simulink model "Water_Treatment_Plant"  (R2026a)
settings: Solver=ode4  StopTime=P.sim.defaultStopTime_s  FixedStep=P.sim.baseStep_s
undefined symbols (not defined in the file): P
settings Model: Creator=jonat  LastModifiedBy=jonat

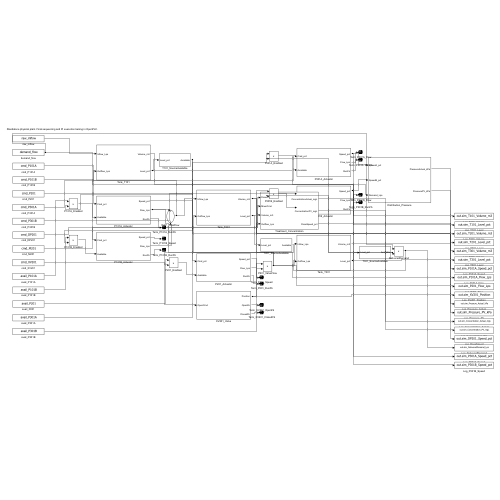
[thumbnail: Simulink's stored preview of the top-level diagram]
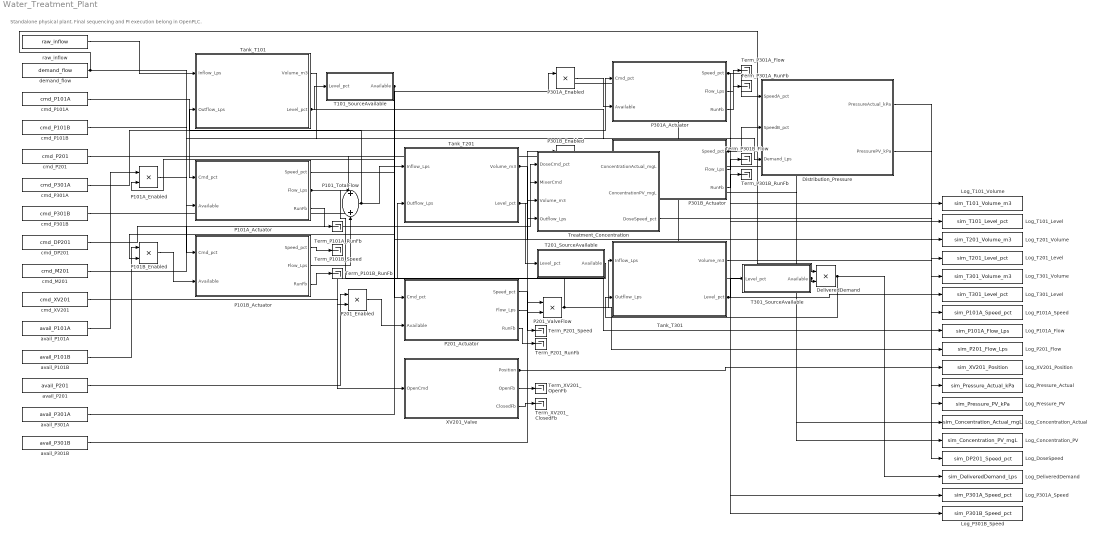
== system Water_Treatment_Plant ==
  note: Standalone physical plant. Final sequencing and PI execution belong in OpenPLC.
  DeliveredDemand : Product  Inputs=**
  Distribution_Pressure : Subsystem
  Log_Concentration_Actual : ToWorkspace  VariableName=sim_Concentration_Actual_mgL  SaveFormat=Timeseries  SampleTime=-1
  Log_Concentration_PV : ToWorkspace  VariableName=sim_Concentration_PV_mgL  SaveFormat=Timeseries  SampleTime=-1
  Log_DeliveredDemand : ToWorkspace  VariableName=sim_DeliveredDemand_Lps  SaveFormat=Timeseries  SampleTime=-1
  Log_DoseSpeed : ToWorkspace  VariableName=sim_DP201_Speed_pct  SaveFormat=Timeseries  SampleTime=-1
  Log_P101A_Flow : ToWorkspace  VariableName=sim_P101A_Flow_Lps  SaveFormat=Timeseries  SampleTime=-1
  Log_P101A_Speed : ToWorkspace  VariableName=sim_P101A_Speed_pct  SaveFormat=Timeseries  SampleTime=-1
  Log_P201_Flow : ToWorkspace  VariableName=sim_P201_Flow_Lps  SaveFormat=Timeseries  SampleTime=-1
  Log_P301A_Speed : ToWorkspace  VariableName=sim_P301A_Speed_pct  SaveFormat=Timeseries  SampleTime=-1
  Log_P301B_Speed : ToWorkspace  VariableName=sim_P301B_Speed_pct  SaveFormat=Timeseries  SampleTime=-1
  Log_Pressure_Actual : ToWorkspace  VariableName=sim_Pressure_Actual_kPa  SaveFormat=Timeseries  SampleTime=-1
  Log_Pressure_PV : ToWorkspace  VariableName=sim_Pressure_PV_kPa  SaveFormat=Timeseries  SampleTime=-1
  Log_T101_Level : ToWorkspace  VariableName=sim_T101_Level_pct  SaveFormat=Timeseries  SampleTime=-1
  Log_T101_Volume : ToWorkspace  VariableName=sim_T101_Volume_m3  SaveFormat=Timeseries  SampleTime=-1
  Log_T201_Level : ToWorkspace  VariableName=sim_T201_Level_pct  SaveFormat=Timeseries  SampleTime=-1
  Log_T201_Volume : ToWorkspace  VariableName=sim_T201_Volume_m3  SaveFormat=Timeseries  SampleTime=-1
  Log_T301_Level : ToWorkspace  VariableName=sim_T301_Level_pct  SaveFormat=Timeseries  SampleTime=-1
  Log_T301_Volume : ToWorkspace  VariableName=sim_T301_Volume_m3  SaveFormat=Timeseries  SampleTime=-1
  Log_XV201_Position : ToWorkspace  VariableName=sim_XV201_Position  SaveFormat=Timeseries  SampleTime=-1
  P101A_Actuator : Subsystem
  P101A_Enabled : Product  Inputs=**
  P101B_Actuator : Subsystem
  P101B_Enabled : Product  Inputs=**
  P101_TotalFlow : Sum
  P201_Actuator : Subsystem
  P201_Enabled : Product  Inputs=**
  P201_ValveFlow : Product  Inputs=**
  P301A_Actuator : Subsystem
  P301A_Enabled : Product  Inputs=**
  P301B_Actuator : Subsystem
  P301B_Enabled : Product  Inputs=**
  T101_SourceAvailable : Subsystem
  T201_SourceAvailable : Subsystem
  T301_SourceAvailable : Subsystem
  Tank_T101 : Subsystem
  Tank_T201 : Subsystem
  Tank_T301 : Subsystem
  Term_P101A_RunFb : Terminator
  Term_P101B_RunFb : Terminator
  Term_P101B_Speed : Terminator
  Term_P201_RunFb : Terminator
  Term_P201_Speed : Terminator
  Term_P301A_Flow : Terminator
  Term_P301A_RunFb : Terminator
  Term_P301B_Flow : Terminator
  Term_P301B_RunFb : Terminator
  Term_XV201_ClosedFb : Terminator
  Term_XV201_OpenFb : Terminator
  Treatment_Concentration : Subsystem
  XV201_Valve : Subsystem
  avail_P101A : FromWorkspace  VariableName=avail_P101A  Interpolate=off  OutputAfterFinalValue=Holding final value
  avail_P101B : FromWorkspace  VariableName=avail_P101B  Interpolate=off  OutputAfterFinalValue=Holding final value
  avail_P201 : FromWorkspace  VariableName=avail_P201  Interpolate=off  OutputAfterFinalValue=Holding final value
  avail_P301A : FromWorkspace  VariableName=avail_P301A  Interpolate=off  OutputAfterFinalValue=Holding final value
  avail_P301B : FromWorkspace  VariableName=avail_P301B  Interpolate=off  OutputAfterFinalValue=Holding final value
  cmd_DP201 : FromWorkspace  VariableName=cmd_DP201  Interpolate=off  OutputAfterFinalValue=Holding final value
  cmd_M201 : FromWorkspace  VariableName=cmd_M201  Interpolate=off  OutputAfterFinalValue=Holding final value
  cmd_P101A : FromWorkspace  VariableName=cmd_P101A  Interpolate=off  OutputAfterFinalValue=Holding final value
  cmd_P101B : FromWorkspace  VariableName=cmd_P101B  Interpolate=off  OutputAfterFinalValue=Holding final value
  cmd_P201 : FromWorkspace  VariableName=cmd_P201  Interpolate=off  OutputAfterFinalValue=Holding final value
  cmd_P301A : FromWorkspace  VariableName=cmd_P301A  Interpolate=off  OutputAfterFinalValue=Holding final value
  cmd_P301B : FromWorkspace  VariableName=cmd_P301B  Interpolate=off  OutputAfterFinalValue=Holding final value
  cmd_XV201 : FromWorkspace  VariableName=cmd_XV201  Interpolate=off  OutputAfterFinalValue=Holding final value
  demand_flow : FromWorkspace  VariableName=demand_flow  Interpolate=off  OutputAfterFinalValue=Holding final value
  raw_inflow : FromWorkspace  VariableName=raw_inflow  Interpolate=off  OutputAfterFinalValue=Holding final value
  wires:
  raw_inflow/1 -> Tank_T101/1(Inflow_Lps)
  Tank_T101/2(Level_pct) -> T101_SourceAvailable/1(Level_pct), Log_T101_Level/1
  avail_P101A/1 -> P101A_Enabled/1
  T101_SourceAvailable/1(Available) -> P101A_Enabled/2, P101B_Enabled/2
  avail_P101B/1 -> P101B_Enabled/1
  cmd_P101A/1 -> P101A_Actuator/1(Cmd_pct)
  P101A_Enabled/1 -> P101A_Actuator/2(Available)
  cmd_P101B/1 -> P101B_Actuator/1(Cmd_pct)
  P101B_Enabled/1 -> P101B_Actuator/2(Available)
  P101A_Actuator/2(Flow_Lps) -> P101_TotalFlow/1, Log_P101A_Flow/1
  P101B_Actuator/2(Flow_Lps) -> P101_TotalFlow/2
  P101_TotalFlow/1 -> Tank_T101/2(Outflow_Lps), Tank_T201/1(Inflow_Lps)
  Tank_T201/2(Level_pct) -> T201_SourceAvailable/1(Level_pct), Log_T201_Level/1
  avail_P201/1 -> P201_Enabled/1
  T201_SourceAvailable/1(Available) -> P201_Enabled/2
  cmd_P201/1 -> P201_Actuator/1(Cmd_pct)
  P201_Enabled/1 -> P201_Actuator/2(Available)
  cmd_XV201/1 -> XV201_Valve/1(OpenCmd)
  P201_Actuator/2(Flow_Lps) -> P201_ValveFlow/1
  XV201_Valve/1(Position) -> P201_ValveFlow/2, Log_XV201_Position/1
  P201_ValveFlow/1 -> Tank_T201/2(Outflow_Lps), Tank_T301/1(Inflow_Lps), Treatment_Concentration/4(Outflow_Lps), Log_P201_Flow/1
  cmd_DP201/1 -> Treatment_Concentration/1(DoseCmd_pct)
  cmd_M201/1 -> Treatment_Concentration/2(MixerCmd)
  Tank_T201/1(Volume_m3) -> Treatment_Concentration/3(Volume_m3), Log_T201_Volume/1
  Tank_T301/2(Level_pct) -> T301_SourceAvailable/1(Level_pct), Log_T301_Level/1
  demand_flow/1 -> DeliveredDemand/1, Distribution_Pressure/3(Demand_Lps)
  T301_SourceAvailable/1(Available) -> DeliveredDemand/2, P301A_Enabled/2, P301B_Enabled/2
  DeliveredDemand/1 -> Tank_T301/2(Outflow_Lps), Log_DeliveredDemand/1
  avail_P301A/1 -> P301A_Enabled/1
  avail_P301B/1 -> P301B_Enabled/1
  cmd_P301A/1 -> P301A_Actuator/1(Cmd_pct)
  P301A_Enabled/1 -> P301A_Actuator/2(Available)
  cmd_P301B/1 -> P301B_Actuator/1(Cmd_pct)
  P301B_Enabled/1 -> P301B_Actuator/2(Available)
  P301A_Actuator/1(Speed_pct) -> Distribution_Pressure/1(SpeedA_pct), Log_P301A_Speed/1
  P301B_Actuator/1(Speed_pct) -> Distribution_Pressure/2(SpeedB_pct), Log_P301B_Speed/1
  P101A_Actuator/3(RunFb) -> Term_P101A_RunFb/1
  P101B_Actuator/1(Speed_pct) -> Term_P101B_Speed/1
  P101B_Actuator/3(RunFb) -> Term_P101B_RunFb/1
  P201_Actuator/1(Speed_pct) -> Term_P201_Speed/1
  P201_Actuator/3(RunFb) -> Term_P201_RunFb/1
  P301A_Actuator/2(Flow_Lps) -> Term_P301A_Flow/1
  P301A_Actuator/3(RunFb) -> Term_P301A_RunFb/1
  P301B_Actuator/2(Flow_Lps) -> Term_P301B_Flow/1
  P301B_Actuator/3(RunFb) -> Term_P301B_RunFb/1
  XV201_Valve/2(OpenFb) -> Term_XV201_OpenFb/1
  XV201_Valve/3(ClosedFb) -> Term_XV201_ClosedFb/1
  Tank_T101/1(Volume_m3) -> Log_T101_Volume/1
  Tank_T301/1(Volume_m3) -> Log_T301_Volume/1
  P101A_Actuator/1(Speed_pct) -> Log_P101A_Speed/1
  Distribution_Pressure/1(PressureActual_kPa) -> Log_Pressure_Actual/1
  Distribution_Pressure/2(PressurePV_kPa) -> Log_Pressure_PV/1
  Treatment_Concentration/1(ConcentrationActual_mgL) -> Log_Concentration_Actual/1
  Treatment_Concentration/2(ConcentrationPV_mgL) -> Log_Concentration_PV/1
  Treatment_Concentration/3(DoseSpeed_pct) -> Log_DoseSpeed/1

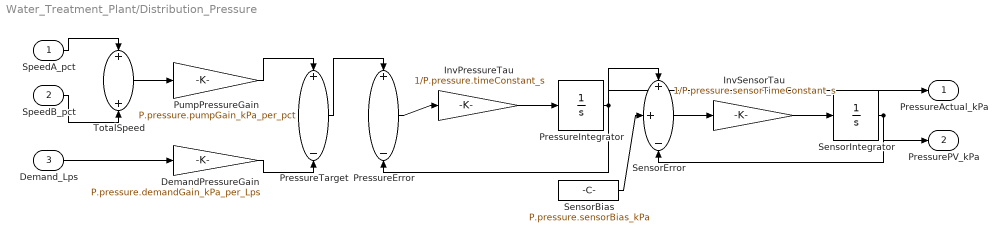
== system Water_Treatment_Plant/Distribution_Pressure ==
  SpeedA_pct : Inport
  SpeedB_pct : Inport  Port=2
  Demand_Lps : Inport  Port=3
  DemandPressureGain : Gain  Gain=P.pressure.demandGain_kPa_per_Lps
  InvPressureTau : Gain  Gain=1/P.pressure.timeConstant_s
  InvSensorTau : Gain  Gain=1/P.pressure.sensorTimeConstant_s
  PressureError : Sum  Inputs=+-
  PressureIntegrator : Integrator  InitialCondition=P.pressure.initial_kPa  LimitOutput=on  UpperSaturationLimit=P.sim.maxPressure_kPa  LowerSaturationLimit=0
  PressureTarget : Sum  Inputs=+-
  PumpPressureGain : Gain  Gain=P.pressure.pumpGain_kPa_per_pct
  SensorBias : Constant  Value=P.pressure.sensorBias_kPa
  SensorError : Sum  Inputs=++-
  SensorIntegrator : Integrator  InitialCondition=P.pressure.initial_kPa  LimitOutput=on  UpperSaturationLimit=P.sim.maxPressure_kPa  LowerSaturationLimit=0
  TotalSpeed : Sum
  PressureActual_kPa : Outport
  PressurePV_kPa : Outport  Port=2
  wires:
  SpeedA_pct/1 -> TotalSpeed/1
  SpeedB_pct/1 -> TotalSpeed/2
  TotalSpeed/1 -> PumpPressureGain/1
  Demand_Lps/1 -> DemandPressureGain/1
  PumpPressureGain/1 -> PressureTarget/1
  DemandPressureGain/1 -> PressureTarget/2
  PressureTarget/1 -> PressureError/1
  PressureIntegrator/1 -> PressureError/2, PressureActual_kPa/1, SensorError/1
  PressureError/1 -> InvPressureTau/1
  InvPressureTau/1 -> PressureIntegrator/1
  SensorBias/1 -> SensorError/2
  SensorIntegrator/1 -> SensorError/3, PressurePV_kPa/1
  SensorError/1 -> InvSensorTau/1
  InvSensorTau/1 -> SensorIntegrator/1

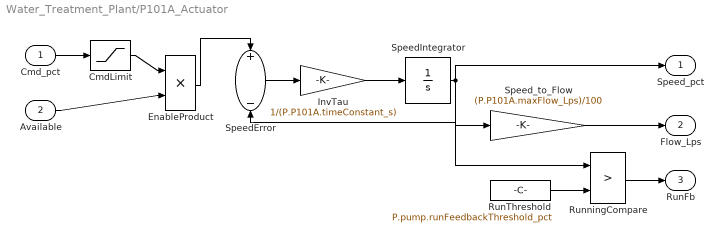
== system Water_Treatment_Plant/P101A_Actuator ==
  Cmd_pct : Inport
  Available : Inport  Port=2
  CmdLimit : Saturate  UpperLimit=100  LowerLimit=0
  EnableProduct : Product  Inputs=**
  InvTau : Gain  Gain=1/(P.P101A.timeConstant_s)
  RunThreshold : Constant  Value=P.pump.runFeedbackThreshold_pct
  RunningCompare : RelationalOperator  Operator=>  OutDataTypeStr=boolean  RndMeth=Simplest  InputSameDT=off
  SpeedError : Sum  Inputs=+-
  SpeedIntegrator : Integrator  LimitOutput=on  UpperSaturationLimit=100  LowerSaturationLimit=0
  Speed_to_Flow : Gain  Gain=(P.P101A.maxFlow_Lps)/100
  Speed_pct : Outport
  Flow_Lps : Outport  Port=2
  RunFb : Outport  Port=3
  wires:
  Cmd_pct/1 -> CmdLimit/1
  CmdLimit/1 -> EnableProduct/1
  Available/1 -> EnableProduct/2
  EnableProduct/1 -> SpeedError/1
  SpeedIntegrator/1 -> SpeedError/2, Speed_pct/1, Speed_to_Flow/1, RunningCompare/1
  SpeedError/1 -> InvTau/1
  InvTau/1 -> SpeedIntegrator/1
  Speed_to_Flow/1 -> Flow_Lps/1
  RunThreshold/1 -> RunningCompare/2
  RunningCompare/1 -> RunFb/1

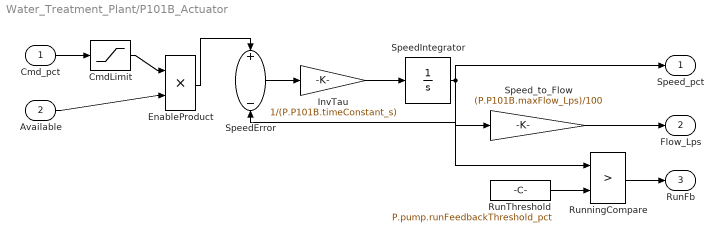
== system Water_Treatment_Plant/P101B_Actuator ==
  Cmd_pct : Inport
  Available : Inport  Port=2
  CmdLimit : Saturate  UpperLimit=100  LowerLimit=0
  EnableProduct : Product  Inputs=**
  InvTau : Gain  Gain=1/(P.P101B.timeConstant_s)
  RunThreshold : Constant  Value=P.pump.runFeedbackThreshold_pct
  RunningCompare : RelationalOperator  Operator=>  OutDataTypeStr=boolean  RndMeth=Simplest  InputSameDT=off
  SpeedError : Sum  Inputs=+-
  SpeedIntegrator : Integrator  LimitOutput=on  UpperSaturationLimit=100  LowerSaturationLimit=0
  Speed_to_Flow : Gain  Gain=(P.P101B.maxFlow_Lps)/100
  Speed_pct : Outport
  Flow_Lps : Outport  Port=2
  RunFb : Outport  Port=3
  wires:
  Cmd_pct/1 -> CmdLimit/1
  CmdLimit/1 -> EnableProduct/1
  Available/1 -> EnableProduct/2
  EnableProduct/1 -> SpeedError/1
  SpeedIntegrator/1 -> SpeedError/2, Speed_pct/1, Speed_to_Flow/1, RunningCompare/1
  SpeedError/1 -> InvTau/1
  InvTau/1 -> SpeedIntegrator/1
  Speed_to_Flow/1 -> Flow_Lps/1
  RunThreshold/1 -> RunningCompare/2
  RunningCompare/1 -> RunFb/1

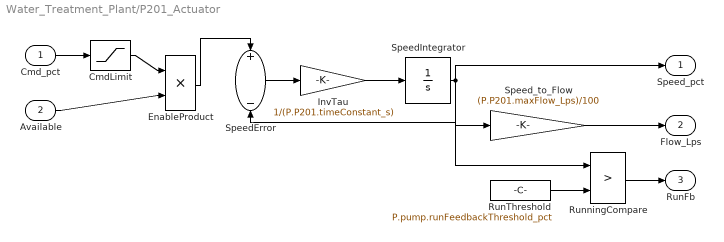
== system Water_Treatment_Plant/P201_Actuator ==
  Cmd_pct : Inport
  Available : Inport  Port=2
  CmdLimit : Saturate  UpperLimit=100  LowerLimit=0
  EnableProduct : Product  Inputs=**
  InvTau : Gain  Gain=1/(P.P201.timeConstant_s)
  RunThreshold : Constant  Value=P.pump.runFeedbackThreshold_pct
  RunningCompare : RelationalOperator  Operator=>  OutDataTypeStr=boolean  RndMeth=Simplest  InputSameDT=off
  SpeedError : Sum  Inputs=+-
  SpeedIntegrator : Integrator  LimitOutput=on  UpperSaturationLimit=100  LowerSaturationLimit=0
  Speed_to_Flow : Gain  Gain=(P.P201.maxFlow_Lps)/100
  Speed_pct : Outport
  Flow_Lps : Outport  Port=2
  RunFb : Outport  Port=3
  wires:
  Cmd_pct/1 -> CmdLimit/1
  CmdLimit/1 -> EnableProduct/1
  Available/1 -> EnableProduct/2
  EnableProduct/1 -> SpeedError/1
  SpeedIntegrator/1 -> SpeedError/2, Speed_pct/1, Speed_to_Flow/1, RunningCompare/1
  SpeedError/1 -> InvTau/1
  InvTau/1 -> SpeedIntegrator/1
  Speed_to_Flow/1 -> Flow_Lps/1
  RunThreshold/1 -> RunningCompare/2
  RunningCompare/1 -> RunFb/1

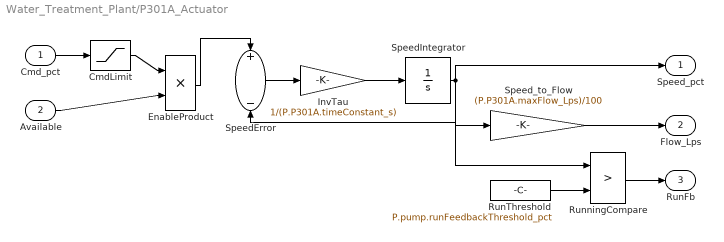
== system Water_Treatment_Plant/P301A_Actuator ==
  Cmd_pct : Inport
  Available : Inport  Port=2
  CmdLimit : Saturate  UpperLimit=100  LowerLimit=0
  EnableProduct : Product  Inputs=**
  InvTau : Gain  Gain=1/(P.P301A.timeConstant_s)
  RunThreshold : Constant  Value=P.pump.runFeedbackThreshold_pct
  RunningCompare : RelationalOperator  Operator=>  OutDataTypeStr=boolean  RndMeth=Simplest  InputSameDT=off
  SpeedError : Sum  Inputs=+-
  SpeedIntegrator : Integrator  LimitOutput=on  UpperSaturationLimit=100  LowerSaturationLimit=0
  Speed_to_Flow : Gain  Gain=(P.P301A.maxFlow_Lps)/100
  Speed_pct : Outport
  Flow_Lps : Outport  Port=2
  RunFb : Outport  Port=3
  wires:
  Cmd_pct/1 -> CmdLimit/1
  CmdLimit/1 -> EnableProduct/1
  Available/1 -> EnableProduct/2
  EnableProduct/1 -> SpeedError/1
  SpeedIntegrator/1 -> SpeedError/2, Speed_pct/1, Speed_to_Flow/1, RunningCompare/1
  SpeedError/1 -> InvTau/1
  InvTau/1 -> SpeedIntegrator/1
  Speed_to_Flow/1 -> Flow_Lps/1
  RunThreshold/1 -> RunningCompare/2
  RunningCompare/1 -> RunFb/1

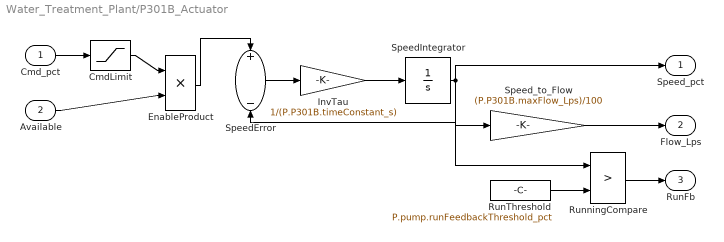
== system Water_Treatment_Plant/P301B_Actuator ==
  Cmd_pct : Inport
  Available : Inport  Port=2
  CmdLimit : Saturate  UpperLimit=100  LowerLimit=0
  EnableProduct : Product  Inputs=**
  InvTau : Gain  Gain=1/(P.P301B.timeConstant_s)
  RunThreshold : Constant  Value=P.pump.runFeedbackThreshold_pct
  RunningCompare : RelationalOperator  Operator=>  OutDataTypeStr=boolean  RndMeth=Simplest  InputSameDT=off
  SpeedError : Sum  Inputs=+-
  SpeedIntegrator : Integrator  LimitOutput=on  UpperSaturationLimit=100  LowerSaturationLimit=0
  Speed_to_Flow : Gain  Gain=(P.P301B.maxFlow_Lps)/100
  Speed_pct : Outport
  Flow_Lps : Outport  Port=2
  RunFb : Outport  Port=3
  wires:
  Cmd_pct/1 -> CmdLimit/1
  CmdLimit/1 -> EnableProduct/1
  Available/1 -> EnableProduct/2
  EnableProduct/1 -> SpeedError/1
  SpeedIntegrator/1 -> SpeedError/2, Speed_pct/1, Speed_to_Flow/1, RunningCompare/1
  SpeedError/1 -> InvTau/1
  InvTau/1 -> SpeedIntegrator/1
  Speed_to_Flow/1 -> Flow_Lps/1
  RunThreshold/1 -> RunningCompare/2
  RunningCompare/1 -> RunFb/1

== system Water_Treatment_Plant/T101_SourceAvailable ==
  Level_pct : Inport
  Compare : RelationalOperator  Operator=>  OutDataTypeStr=boolean  RndMeth=Simplest  InputSameDT=off
  MinimumLevel : Constant  Value=P.tank.minimumSourceLevel_pct
  Available : Outport
  wires:
  Level_pct/1 -> Compare/1
  MinimumLevel/1 -> Compare/2
  Compare/1 -> Available/1

== system Water_Treatment_Plant/T201_SourceAvailable ==
  Level_pct : Inport
  Compare : RelationalOperator  Operator=>  OutDataTypeStr=boolean  RndMeth=Simplest  InputSameDT=off
  MinimumLevel : Constant  Value=P.tank.minimumSourceLevel_pct
  Available : Outport
  wires:
  Level_pct/1 -> Compare/1
  MinimumLevel/1 -> Compare/2
  Compare/1 -> Available/1

== system Water_Treatment_Plant/T301_SourceAvailable ==
  Level_pct : Inport
  Compare : RelationalOperator  Operator=>  OutDataTypeStr=boolean  RndMeth=Simplest  InputSameDT=off
  MinimumLevel : Constant  Value=P.tank.minimumSourceLevel_pct
  Available : Outport
  wires:
  Level_pct/1 -> Compare/1
  MinimumLevel/1 -> Compare/2
  Compare/1 -> Available/1

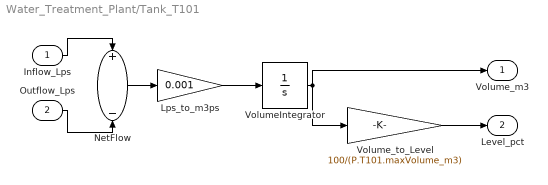
== system Water_Treatment_Plant/Tank_T101 ==
  Inflow_Lps : Inport
  Outflow_Lps : Inport  Port=2
  Lps_to_m3ps : Gain  Gain=0.001
  NetFlow : Sum  Inputs=+-
  VolumeIntegrator : Integrator  InitialCondition=P.T101.initialVolume_m3  LimitOutput=on  UpperSaturationLimit=P.T101.maxVolume_m3  LowerSaturationLimit=0
  Volume_to_Level : Gain  Gain=100/(P.T101.maxVolume_m3)
  Volume_m3 : Outport
  Level_pct : Outport  Port=2
  wires:
  Inflow_Lps/1 -> NetFlow/1
  Outflow_Lps/1 -> NetFlow/2
  NetFlow/1 -> Lps_to_m3ps/1
  Lps_to_m3ps/1 -> VolumeIntegrator/1
  VolumeIntegrator/1 -> Volume_m3/1, Volume_to_Level/1
  Volume_to_Level/1 -> Level_pct/1

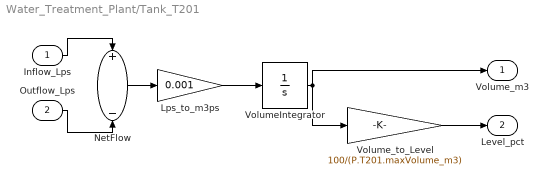
== system Water_Treatment_Plant/Tank_T201 ==
  Inflow_Lps : Inport
  Outflow_Lps : Inport  Port=2
  Lps_to_m3ps : Gain  Gain=0.001
  NetFlow : Sum  Inputs=+-
  VolumeIntegrator : Integrator  InitialCondition=P.T201.initialVolume_m3  LimitOutput=on  UpperSaturationLimit=P.T201.maxVolume_m3  LowerSaturationLimit=0
  Volume_to_Level : Gain  Gain=100/(P.T201.maxVolume_m3)
  Volume_m3 : Outport
  Level_pct : Outport  Port=2
  wires:
  Inflow_Lps/1 -> NetFlow/1
  Outflow_Lps/1 -> NetFlow/2
  NetFlow/1 -> Lps_to_m3ps/1
  Lps_to_m3ps/1 -> VolumeIntegrator/1
  VolumeIntegrator/1 -> Volume_m3/1, Volume_to_Level/1
  Volume_to_Level/1 -> Level_pct/1

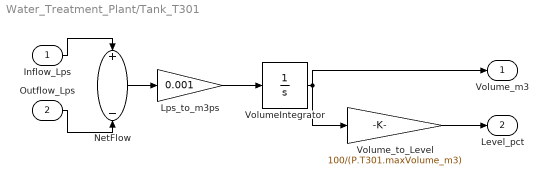
== system Water_Treatment_Plant/Tank_T301 ==
  Inflow_Lps : Inport
  Outflow_Lps : Inport  Port=2
  Lps_to_m3ps : Gain  Gain=0.001
  NetFlow : Sum  Inputs=+-
  VolumeIntegrator : Integrator  InitialCondition=P.T301.initialVolume_m3  LimitOutput=on  UpperSaturationLimit=P.T301.maxVolume_m3  LowerSaturationLimit=0
  Volume_to_Level : Gain  Gain=100/(P.T301.maxVolume_m3)
  Volume_m3 : Outport
  Level_pct : Outport  Port=2
  wires:
  Inflow_Lps/1 -> NetFlow/1
  Outflow_Lps/1 -> NetFlow/2
  NetFlow/1 -> Lps_to_m3ps/1
  Lps_to_m3ps/1 -> VolumeIntegrator/1
  VolumeIntegrator/1 -> Volume_m3/1, Volume_to_Level/1
  Volume_to_Level/1 -> Level_pct/1

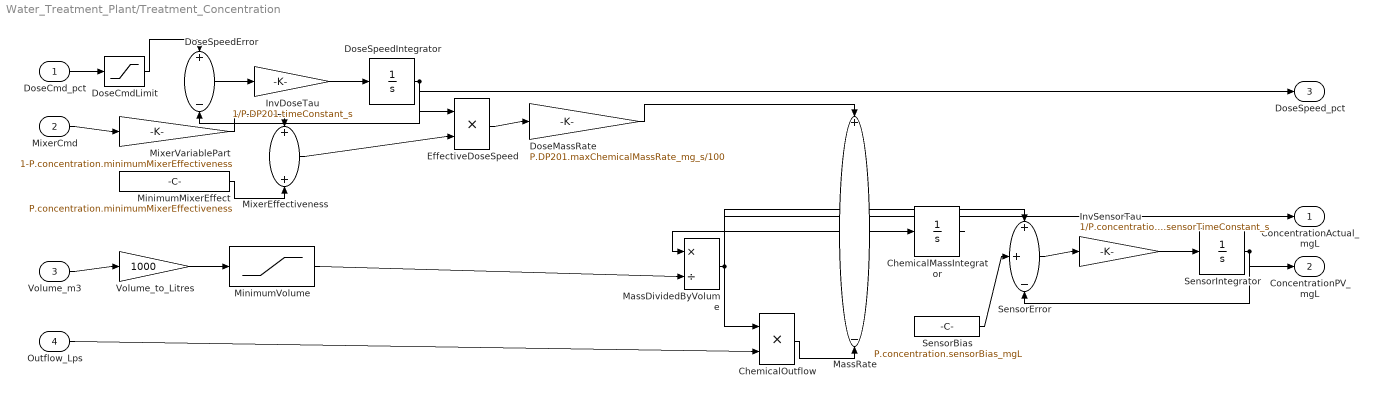
== system Water_Treatment_Plant/Treatment_Concentration ==
  DoseCmd_pct : Inport
  MixerCmd : Inport  Port=2
  Volume_m3 : Inport  Port=3
  Outflow_Lps : Inport  Port=4
  ChemicalMassIntegrator : Integrator  InitialCondition=P.T201.initialConcentration_mgL*P.T201.initialVolume_m3*1000  LimitOutput=on  UpperSaturationLimit=P.T201.maxVolume_m3*1000*P.concentration.maxPhysical_mgL  LowerSaturationLimit=0
  ChemicalOutflow : Product  Inputs=**
  DoseCmdLimit : Saturate  UpperLimit=100  LowerLimit=0
  DoseMassRate : Gain  Gain=P.DP201.maxChemicalMassRate_mg_s/100
  DoseSpeedError : Sum  Inputs=+-
  DoseSpeedIntegrator : Integrator  LimitOutput=on  UpperSaturationLimit=100  LowerSaturationLimit=0
  EffectiveDoseSpeed : Product  Inputs=**
  InvDoseTau : Gain  Gain=1/P.DP201.timeConstant_s
  InvSensorTau : Gain  Gain=1/P.concentration.sensorTimeConstant_s
  MassDividedByVolume : Product  Inputs=*/
  MassRate : Sum  Inputs=+-
  MinimumMixerEffect : Constant  Value=P.concentration.minimumMixerEffectiveness
  MinimumVolume : Saturate  UpperLimit=P.T201.maxVolume_m3*1000  LowerLimit=100
  MixerEffectiveness : Sum
  MixerVariablePart : Gain  Gain=1-P.concentration.minimumMixerEffectiveness
  SensorBias : Constant  Value=P.concentration.sensorBias_mgL
  SensorError : Sum  Inputs=++-
  SensorIntegrator : Integrator  InitialCondition=P.T201.initialConcentration_mgL  LimitOutput=on  UpperSaturationLimit=P.concentration.maxPhysical_mgL  LowerSaturationLimit=0
  Volume_to_Litres : Gain  Gain=1000
  ConcentrationActual_mgL : Outport
  ConcentrationPV_mgL : Outport  Port=2
  DoseSpeed_pct : Outport  Port=3
  wires:
  DoseCmd_pct/1 -> DoseCmdLimit/1
  DoseCmdLimit/1 -> DoseSpeedError/1
  DoseSpeedIntegrator/1 -> DoseSpeedError/2, DoseSpeed_pct/1, EffectiveDoseSpeed/1
  DoseSpeedError/1 -> InvDoseTau/1
  InvDoseTau/1 -> DoseSpeedIntegrator/1
  MixerCmd/1 -> MixerVariablePart/1
  MixerVariablePart/1 -> MixerEffectiveness/1
  MinimumMixerEffect/1 -> MixerEffectiveness/2
  MixerEffectiveness/1 -> EffectiveDoseSpeed/2
  EffectiveDoseSpeed/1 -> DoseMassRate/1
  Volume_m3/1 -> Volume_to_Litres/1
  Volume_to_Litres/1 -> MinimumVolume/1
  ChemicalMassIntegrator/1 -> MassDividedByVolume/1
  MinimumVolume/1 -> MassDividedByVolume/2
  MassDividedByVolume/1 -> ChemicalOutflow/1, ConcentrationActual_mgL/1, SensorError/1
  Outflow_Lps/1 -> ChemicalOutflow/2
  DoseMassRate/1 -> MassRate/1
  ChemicalOutflow/1 -> MassRate/2
  MassRate/1 -> ChemicalMassIntegrator/1
  SensorBias/1 -> SensorError/2
  SensorIntegrator/1 -> SensorError/3, ConcentrationPV_mgL/1
  SensorError/1 -> InvSensorTau/1
  InvSensorTau/1 -> SensorIntegrator/1

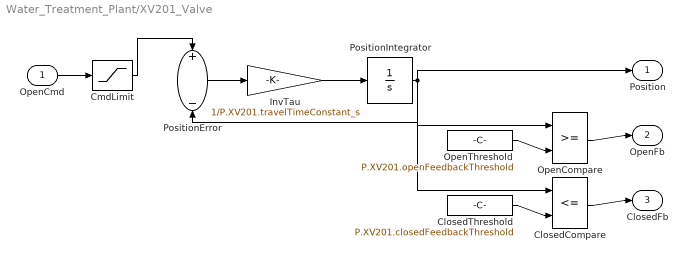
== system Water_Treatment_Plant/XV201_Valve ==
  OpenCmd : Inport
  ClosedCompare : RelationalOperator  Operator=<=  OutDataTypeStr=boolean  RndMeth=Simplest  InputSameDT=off
  ClosedThreshold : Constant  Value=P.XV201.closedFeedbackThreshold
  CmdLimit : Saturate  UpperLimit=1  LowerLimit=0
  InvTau : Gain  Gain=1/P.XV201.travelTimeConstant_s
  OpenCompare : RelationalOperator  OutDataTypeStr=boolean  RndMeth=Simplest  InputSameDT=off
  OpenThreshold : Constant  Value=P.XV201.openFeedbackThreshold
  PositionError : Sum  Inputs=+-
  PositionIntegrator : Integrator  LimitOutput=on  UpperSaturationLimit=1  LowerSaturationLimit=0
  Position : Outport
  OpenFb : Outport  Port=2
  ClosedFb : Outport  Port=3
  wires:
  OpenCmd/1 -> CmdLimit/1
  CmdLimit/1 -> PositionError/1
  PositionIntegrator/1 -> PositionError/2, Position/1, OpenCompare/1, ClosedCompare/1
  PositionError/1 -> InvTau/1
  InvTau/1 -> PositionIntegrator/1
  OpenThreshold/1 -> OpenCompare/2
  OpenCompare/1 -> OpenFb/1
  ClosedThreshold/1 -> ClosedCompare/2
  ClosedCompare/1 -> ClosedFb/1
